simulink model "Grading_System"  (R2021a)
settings: Solver=FixedStepDiscrete  StartTime=0.0  StopTime=10.0  RelTol=1e-3
settings Model: Creator=Dell  LastModifiedBy=Dell
settings OptimizationCC: DefaultParameterBehavior=Inlined  EnhancedBackFolding=on  PassReuseOutputArgsAs=Individual arguments  ZeroExternalMemoryAtStartup=off  ZeroInternalMemoryAtStartup=off  OptimizeBlockOrder=speed  DifferentSizesBufferReuse=on  OptimizationCustomize=off  EfficientTunableParamExpr=on
settings DebuggingCC: ParameterTunabilityLossMsg=error
settings SFSimCC: MATLABDynamicMemAlloc=off
settings RTWCC: SystemTargetFile=ert.tlc  GenCodeOnly=on  TemplateMakefile=ert_default_tmf  GenerateReport=on  IncludeHyperlinkInReport=on  LaunchReport=on  GenerateTraceInfo=on
settings CodeAppCC: ForceParamTrailComments=on  IgnoreCustomStorageClasses=off  OperatorAnnotations=on  SimulinkDataObjDesc=on  SFDataObjDesc=on  InsertBlockDesc=on
settings ERTTargetCC: TargetLangStandard=C99 (ISO)  GenerateSampleERTMain=on  InlinedParameterPlacement=NonHierarchical  ERTCustomFileTemplate=example_file_process.tlc

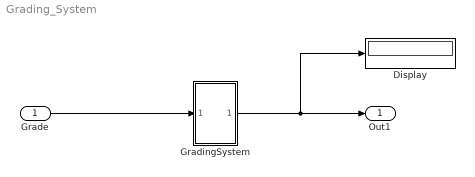
== system Grading_System ==
  Grade : Inport  OutDataTypeStr=uint8
  Display : Display
  GradingSystem : Subsystem  TreatAsAtomicUnit=on
      settings: RTWFcnNameOpts=Use subsystem name  RTWFileNameOpts=Use subsystem name
  Out1 : Outport  OutDataTypeStr=string
  wires:
  GradingSystem/1(Out1) -> Out1/1, Display/1
  Grade/1 -> GradingSystem/1(Grade)

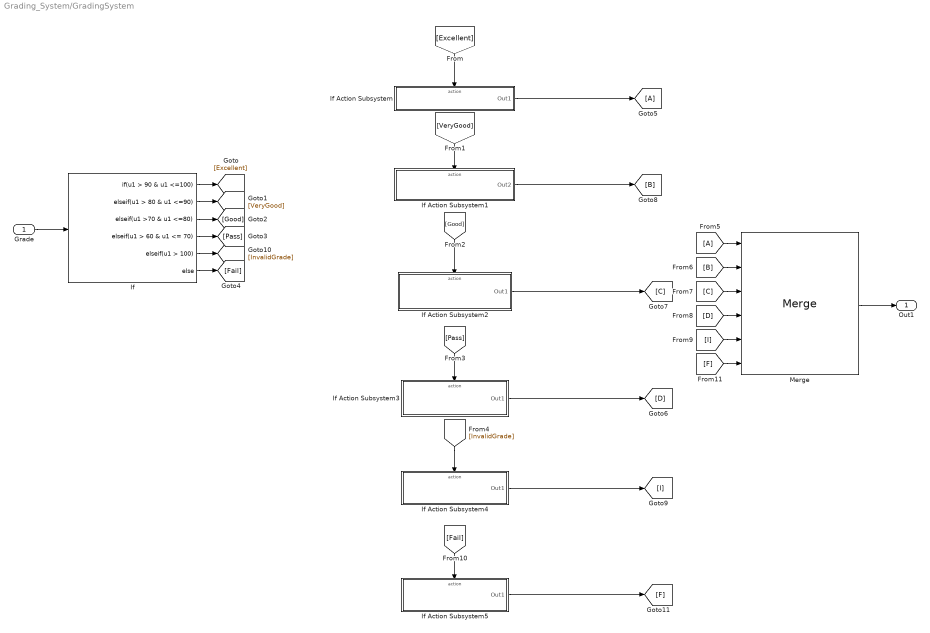
== system Grading_System/GradingSystem ==
  Grade : Inport
  If : If  IfExpression=u1 > 90 & u1 <=100  ElseIfExpressions=u1 > 80 & u1 <=90, u1 >70 & u1 <=80, u1 > 60 & u1 <= 70,u1 > 100
  If Action Subsystem : Subsystem  TreatAsAtomicUnit=on
  If Action Subsystem1 : Subsystem  TreatAsAtomicUnit=on
  If Action Subsystem2 : Subsystem  TreatAsAtomicUnit=on
  If Action Subsystem3 : Subsystem  TreatAsAtomicUnit=on
  If Action Subsystem4 : Subsystem  TreatAsAtomicUnit=on
  If Action Subsystem5 : Subsystem  TreatAsAtomicUnit=on
  Merge : Merge  Inputs=6
  Out1 : Outport
  wires:
  [I] -> Merge/5
  [B] -> Merge/2
  [A] -> Merge/1
  Merge/1 -> Out1/1
  If/6 -> [Fail]
  [InvalidGrade] -> If Action Subsystem4/Action
  [Pass] -> If Action Subsystem3/Action
  If/5 -> [InvalidGrade]
  [Good] -> If Action Subsystem2/Action
  [D] -> Merge/4
  If Action Subsystem5/1(Out1) -> [F]
  [Excellent] -> If Action Subsystem/Action
  [C] -> Merge/3
  If Action Subsystem4/1(Out1) -> [I]
  If Action Subsystem3/1(Out1) -> [D]
  If/4 -> [Pass]
  [VeryGood] -> If Action Subsystem1/Action
  If/2 -> [VeryGood]
  If Action Subsystem/1(Out1) -> [A]
  [Fail] -> If Action Subsystem5/Action
  If Action Subsystem2/1(Out1) -> [C]
  [F] -> Merge/6
  If/3 -> [Good]
  If/1 -> [Excellent]
  If Action Subsystem1/1(Out2) -> [B]
  Grade/1 -> If/1

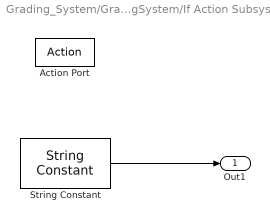
== system Grading_System/GradingSystem/If Action Subsystem ==
  Action Port : ActionPort  InitializeStates=reset  ActionPortLabel=if(u1 > 90 & u1 <=100)
  String Constant : StringConstant  String="\"Distinct\""
  Out1 : Outport  OutDataTypeStr=string
  wires:
  String Constant/1 -> Out1/1

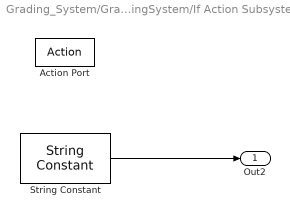
== system Grading_System/GradingSystem/If Action Subsystem1 ==
  Action Port : ActionPort  ActionPortLabel=elseif(u1 > 80 & u1 <=90)
  String Constant : StringConstant  String="\"Very Good\""
  Out2 : Outport  OutDataTypeStr=string
  wires:
  String Constant/1 -> Out2/1

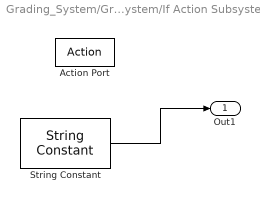
== system Grading_System/GradingSystem/If Action Subsystem2 ==
  Action Port : ActionPort  ActionPortLabel=elseif( u1 >70 & u1 <=80)
  String Constant : StringConstant  String="\"Good\""
  Out1 : Outport  OutDataTypeStr=string
  wires:
  String Constant/1 -> Out1/1

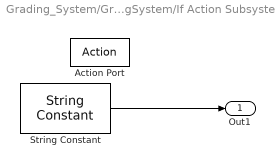
== system Grading_System/GradingSystem/If Action Subsystem3 ==
  Action Port : ActionPort  ActionPortLabel=elseif( u1 > 60 & u1 <= 70)
  String Constant : StringConstant  String="\"Pass\""
  Out1 : Outport  OutDataTypeStr=string
  wires:
  String Constant/1 -> Out1/1

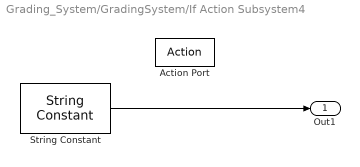
== system Grading_System/GradingSystem/If Action Subsystem4 ==
  Action Port : ActionPort  ActionPortLabel=elseif(u1 > 100)
  String Constant : StringConstant  String="\"Invalid Grade\""
  Out1 : Outport  OutDataTypeStr=string
  wires:
  String Constant/1 -> Out1/1

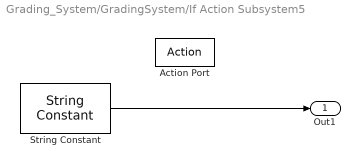
== system Grading_System/GradingSystem/If Action Subsystem5 ==
  Action Port : ActionPort  ActionPortLabel=else
  String Constant : StringConstant  String="\"Fail\""
  Out1 : Outport  OutDataTypeStr=string
  wires:
  String Constant/1 -> Out1/1
